simulink model "controller_Delta3D_feedback"  (R2018b)
settings: Solver=ode45  StartTime=0.0  StopTime=0.5  RelTol=1e-3  EnableMultiTasking=on
values from neighbouring files (symbols this model uses):
  g = 9.81    [project_week_5.m]
  h0 = thetaA_0(1)    [project_week_5.m]
  hm = thetaA_0(1)*0.5    [project_week_5.m]
  I_lower_xx = I_C(4)    [calculate_lagrange.m]    (also in calculate_lagrange_dependent.m; calculate_lagrange_fast.m; project_week_5.m = (1/12)*m_l*L(2)^2)
  I_lower_yy = I_C(5)    [calculate_lagrange.m]    (also in calculate_lagrange_dependent.m; calculate_lagrange_fast.m; project_week_5.m = (1/12)*m_l*L(2)^2)
  I_lower_zz = I_C(6)    [calculate_lagrange.m]    (also in calculate_lagrange_dependent.m; calculate_lagrange_fast.m; project_week_5.m = I_lower_xx/10)
  I_upper_xx = I_C(1)    [calculate_lagrange.m]    (also in calculate_lagrange_dependent.m; calculate_lagrange_fast.m; project_week_5.m = (1/12)*m_u*L(1)^2)
  I_upper_yy = I_C(2)    [calculate_lagrange.m]    (also in calculate_lagrange_dependent.m; calculate_lagrange_fast.m; project_week_5.m = (1/12)*m_u*L(1)^2)
  I_upper_zz = I_C(3)    [calculate_lagrange.m]    (also in calculate_lagrange_dependent.m; calculate_lagrange_fast.m; project_week_5.m = I_upper_xx/10)
  kc = M*wc^2*sqrt(alpha)    [project_week_5.m]
  L = [0.5,1,0.3,0.8]    [plot_inverse.m]    (also in project_week_5.m; project_week_5_boundaries.m = [0.8,1,0.4,0.5]; project_week_5_symbolic.m = [L_u L_l L_e L_b])
  m_l = 0.35    [project_week_5.m]
  m_p = 1    [project_week_5.m]
  m_u = 0.35    [project_week_5.m]
  q0d = q0(ind_d)    [project_week_5.m]
  q0i = q0(ind_i)    [project_week_5.m]
  R_L1_0 = R_L1_t(:,:,1)    [calculate_acceleration.m]    (also in calculate_position.m = R_L0(:,:,1); calculate_position_dep.m = R_L0(:,:,1); calculate_position_fast.m = R_L0(:,:,1); plot_inverse.m = R_A1*rot3D_Rodrigues([0;1;0],thetaL1_y_0))
  R_L2_0 = R_L2_t(:,:,1)    [calculate_acceleration.m]    (also in calculate_position.m = R_L0(:,:,2); calculate_position_dep.m = R_L0(:,:,2); calculate_position_fast.m = R_L0(:,:,2); plot_inverse.m = R_A2*rot3D_Rodrigues([0;1;0],thetaL2_y_0))
  R_L3_0 = R_L3_t(:,:,1)    [calculate_acceleration.m]    (also in calculate_position.m = R_L0(:,:,3); calculate_position_dep.m = R_L0(:,:,3); calculate_position_fast.m = R_L0(:,:,3); plot_inverse.m = R_A3*rot3D_Rodrigues([0;1;0],thetaL3_y_0))
  thetaA_0 = [thetaU1_y_0 ; thetaU2_y_0 ;thetaU3_y_0]    [plot_inverse.m]    (also in project_week_5.m; project_week_5_boundaries.m)
  ti = beta*tz    [project_week_5.m]
  tm = cycleTime    (= 0.35)    [project_week_5.m]
  tp = alpha*tz    [project_week_5.m]
  tz = 1/(wc*sqrt(alpha))    [project_week_5.m]
settings Model: Creator=wouterh  LastModifiedBy=sinai
settings DataIOCC: LimitDataPoints=on  SaveFormat=Array  SignalLoggingSaveFormat=ModelDataLogs
settings OptimizationCC: ExpressionDepthLimit=2147483647  InitFltsAndDblsToZero=on  LifeSpan=inf
settings DebuggingCC: UnderspecifiedInitializationDetection=Classic  MergeDetectMultiDrivingBlocksExec=none  SolverPrmCheckMsg=warning  FcnCallInpInsideContextMsg=warning  StateNameClashWarn=warning  LibraryContextMissingDiagnostic=none  SFUnexpectedBacktrackingDiag=warning  SFNoUnconditionalDefaultTransitionDiag=warning  SFExecutionAtInitializationDiag=none
settings HardwareCC: ProdBitPerPointer=32  ProdBitPerSizeT=32  ProdBitPerPtrDiffT=32  ProdLargestAtomicFloat=None  ProdIntDivRoundTo=Undefined  ProdEndianess=Unspecified  ProdWordSize=32  ProdHWDeviceType=32-bit Generic
settings ModelReferenceCC: PropagateSignalLabelsOutOfModel=off
settings SFSimCC: SimUseLocalCustomCode=off
settings RTWCC: RTWUseLocalCustomCode=off
settings CodeAppCC: StateflowObjectComments=on
settings GRTTargetCC: TargetLangStandard=C89/C90 (ANSI)  CombineOutputUpdateFcns=off  GRTInterface=on
settings ConfigComp: CovMetricSettings=dw  CovHtmlReporting=on  CovSaveCumulativeToWorkspaceVar=on  CovSaveSingleToWorkspaceVar=on  CovExternalEMLEnable=off

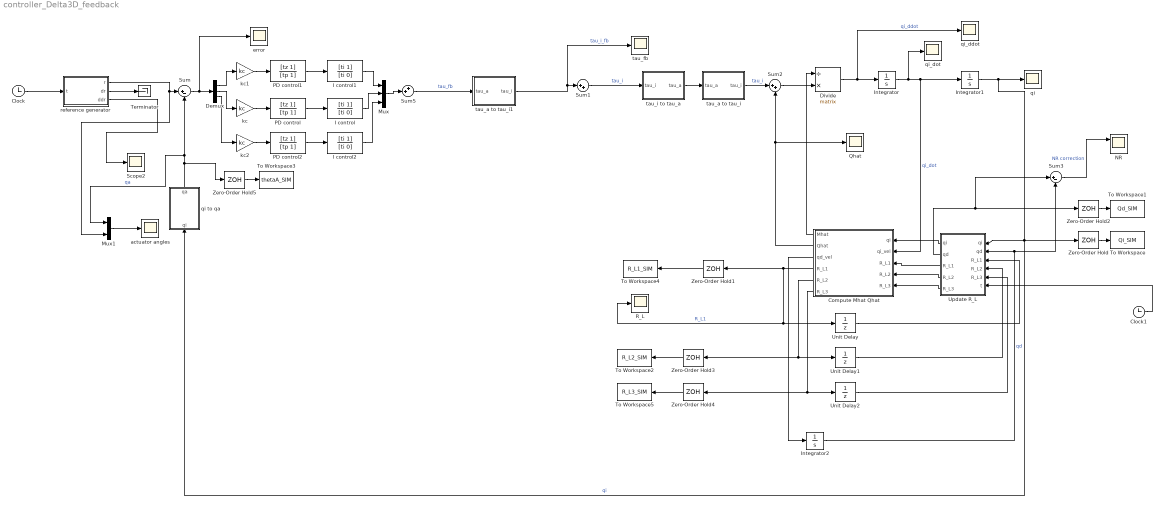
== system controller_Delta3D_feedback ==
  Clock : Clock
  Clock1 : Clock
  Compute Mhat Qhat : MATLAB Function  TreatAsAtomicUnit=on
  Demux : Demux  Outputs=3
  Divide : Product  Inputs=/*  Multiplication=Matrix(*)
  I control : TransferFcn  Numerator=[ti 1]  Denominator=[ti 0]
  I control1 : TransferFcn  Numerator=[ti 1]  Denominator=[ti 0]
  I control2 : TransferFcn  Numerator=[ti 1]  Denominator=[ti 0]
  Integrator : Integrator
  Integrator1 : Integrator  InitialCondition=q0i
  Integrator2 : Integrator  InitialCondition=q0d
  Mux : Mux  Inputs=3
  Mux1 : Mux  Inputs=2
  NR : Scope  NumInputPorts=2
  PD control : TransferFcn  Numerator=[tz 1]  Denominator=[tp 1]
  PD control1 : TransferFcn  Numerator=[tz 1]  Denominator=[tp 1]
  PD control2 : TransferFcn  Numerator=[tz 1]  Denominator=[tp 1]
  Qhat : Scope
  R_L : Scope
  Scope2 : Scope
  Sum : Sum  Inputs=|+-
  Sum1 : Sum  Inputs=|++
  Sum2 : Sum  Inputs=|++
  Sum3 : Sum  Inputs=|+-
  Sum5 : Sum  Inputs=++|
  Terminator : Terminator
  To Workspace : ToWorkspace  VariableName=Qi_SIM  SaveFormat=Timeseries  SampleTime=-1
  To Workspace1 : ToWorkspace  VariableName=Qd_SIM  SaveFormat=Timeseries  SampleTime=-1
  To Workspace2 : ToWorkspace  VariableName=R_L2_SIM  SaveFormat=Timeseries  SampleTime=-1
  To Workspace3 : ToWorkspace  VariableName=thetaA_SIM  SaveFormat=Timeseries  SampleTime=-1
  To Workspace4 : ToWorkspace  VariableName=R_L1_SIM  SaveFormat=Timeseries  SampleTime=-1
  To Workspace5 : ToWorkspace  VariableName=R_L3_SIM  SaveFormat=Timeseries  SampleTime=-1
  Unit Delay : UnitDelay  InitialCondition=R_L1_0  SampleTime=-1
  Unit Delay1 : UnitDelay  InitialCondition=R_L2_0  SampleTime=-1
  Unit Delay2 : UnitDelay  InitialCondition=R_L3_0  SampleTime=-1
  Update R_L : MATLAB Function  TreatAsAtomicUnit=on  SystemSampleTime=0.001
  Zero-Order Hold{,1..5} (6 alike) : ZeroOrderHold  SampleTime=0.02
  actuator angles : Scope
  error : Scope
  kc : Gain  Gain=kc
  kc1 : Gain  Gain=kc
  kc2 : Gain  Gain=kc
  qi : Scope
  qi to qa : MATLAB Function  TreatAsAtomicUnit=on
  qi_ddot : Scope
  qi_dot : Scope
  reference generator : MATLAB Function  TreatAsAtomicUnit=on
  tau_a to tau_i : MATLAB Function  TreatAsAtomicUnit=on
  tau_a to tau_i1 : MATLAB Function  TreatAsAtomicUnit=on
  tau_fb : Scope
  tau_i to tau_a : MATLAB Function  TreatAsAtomicUnit=on
  wires:
  Clock/1 -> reference generator/1(t)
  reference generator/2(dr) -> Terminator/1
  reference generator/3(ddr) -> Scope2/1
  Sum/1 -> Demux/1, error/1
  PD control/1 -> I control/1
  Divide/1 -> qi_ddot/1, Integrator/1  "qi_ddot"
  Integrator/1 -> qi_dot/1, Integrator1/1, Compute Mhat Qhat/2(qi_vel)  "qi_dot"
  Integrator1/1 -> qi to qa/1(qi), Update R_L/1("qi "), Zero-Order Hold/1, qi/1  "qi"
  Compute Mhat Qhat/1(Mhat) -> Divide/1
  PD control1/1 -> I control1/1
  I control/1 -> Mux/2
  I control1/1 -> Mux/1
  Mux/1 -> Sum5/2
  Sum5/1 -> tau_a to tau_i1/1(tau_a)  "tau_fb"
  Mux1/1 -> actuator angles/1
  Compute Mhat Qhat/3(qd_vel) -> Integrator2/1
  kc1/1 -> PD control1/1
  Demux/1 -> kc1/1
  Demux/2 -> kc/1
  kc/1 -> PD control/1
  reference generator/1(r) -> Mux1/2, Sum/1
  Zero-Order Hold/1 -> To Workspace/1
  Zero-Order Hold2/1 -> To Workspace1/1
  Unit Delay/1 -> Update R_L/3("R_L1 ")
  Compute Mhat Qhat/4(R_L1) -> Zero-Order Hold1/1, R_L/1, Unit Delay/1  "R_L1"
  I control2/1 -> Mux/3
  kc2/1 -> PD control2/1
  PD control2/1 -> I control2/1
  Demux/3 -> kc2/1
  Sum2/1 -> Divide/2
  tau_a to tau_i/1(tau_i) -> Sum2/1  "tau_i"
  qi to qa/1(qa) -> Mux1/1, Sum/2, Zero-Order Hold5/1  "qa"
  Compute Mhat Qhat/5(R_L2) -> Zero-Order Hold3/1, Unit Delay1/1
  Compute Mhat Qhat/6(R_L3) -> Unit Delay2/1, Zero-Order Hold4/1
  Unit Delay2/1 -> Update R_L/5("R_L3 ")
  tau_i to tau_a/1(tau_a) -> tau_a to tau_i/1(tau_a)
  Sum1/1 -> tau_i to tau_a/1(tau_i)  "tau_i"
  tau_a to tau_i1/1(tau_i) -> tau_fb/1, Sum1/1  "tau_i_fb"
  Unit Delay1/1 -> Update R_L/4("R_L2 ")
  Zero-Order Hold1/1 -> To Workspace4/1
  Zero-Order Hold3/1 -> To Workspace2/1
  Update R_L/1(qi) -> Compute Mhat Qhat/1(qi)
  Integrator2/1 -> Sum3/2, Update R_L/2("qd ")  "qd"
  Update R_L/2(qd) -> Sum3/1, Zero-Order Hold2/1
  Update R_L/3(R_L1) -> Compute Mhat Qhat/3("R_L1 ")
  Update R_L/4(R_L2) -> Compute Mhat Qhat/4("R_L2 ")
  Update R_L/5(R_L3) -> Compute Mhat Qhat/5("R_L3 ")
  Zero-Order Hold4/1 -> To Workspace5/1
  Clock1/1 -> Update R_L/6(t)
  Zero-Order Hold5/1 -> To Workspace3/1
  Sum3/1 -> NR/1  "NR correction"
  Compute Mhat Qhat/2(Qhat) -> Qhat/1, Sum2/2

== matlab function controller_Delta3D_feedback/Compute Mhat Qhat ==
  data: qi input; qi_vel input; R_L1 input; R_L2 input; R_L3 input; Mhat output; Qhat output; m_u parameter; m_p parameter; m_l parameter; L parameter; g parameter; I_upper_xx parameter; I_upper_yy parameter; I_upper_zz parameter; I_lower_xx parameter; I_lower_yy parameter; I_lower_zz parameter; thetaA_0 parameter; qd_vel output; R_L1 output; R_L2 output; R_L3 output
function [Mhat, Qhat,qd_vel,R_L1,R_L2,R_L3] = ...
    computeMhatQhat(qi,qi_vel,R_L1,R_L2,R_L3,...
        m_u, m_p, m_l, L, g,...
        I_upper_xx, I_upper_yy, I_upper_zz,...
        I_lower_xx, I_lower_yy, I_lower_zz,...
        thetaA_0)
% Compute dynamics for the system 
% Assume the model is perfect, so this is a copy past of M_Q_AC_model

%Pre-initialise for Simulink
Mhat=zeros(9,9);
Qhat=zeros(9,1);
qd_vel=zeros(33,1);

% independent and dependent co-ordinate indices
ind_i=[7:9,19:21,31:33]';
% ind_d=(1:42)'; 
% ind_d(ind_i)=[]; % remove independent co-ordinates -> doesn't work in Simulink
ind_d = [1:6,10:18,22:30,34:42]';

%% Parameters
L_u=L(1);
L_l=L(2);
L_e=L(3);
L_b=L(4);

thetaA1 = qi(1)/(+3^(1/2)/2) + thetaA_0(1); 
thetaA2 = qi(4)/(-3^(1/2)/2) + thetaA_0(2); 
thetaA3 = qi(8); 
   
% upper rotation matrices
R_A1=rot3D_Rodrigues([0;0;1],-2*pi/3); % constant
R_U1=R_A1*rot3D_Rodrigues([0;1;0],thetaA1); 

R_A2=rot3D_Rodrigues([0;0;1],2*pi/3); % constant
R_U2=R_A2*rot3D_Rodrigues([0;1;0],thetaA2); 

R_A3=rot3D_Rodrigues([0;0;1],0); % constant
R_U3=R_A3*rot3D_Rodrigues([0;1;0],thetaA3); 

% R_L1
rL1_1_1 = R_L1(1,1); rL1_1_2 = R_L1(1,2); rL1_1_3 = R_L1(1,3);
rL1_2_1 = R_L1(2,1); rL1_2_2 = R_L1(2,2); rL1_2_3 = R_L1(2,3);
rL1_3_1 = R_L1(3,1); rL1_3_2 = R_L1(3,2); rL1_3_3 = R_L1(3,3);

% R_L2
rL2_1_1 = R_L2(1,1); rL2_1_2 = R_L2(1,2); rL2_1_3 = R_L2(1,3);
rL2_2_1 = R_L2(2,1); rL2_2_2 = R_L2(2,2); rL2_2_3 = R_L2(2,3);
rL2_3_1 = R_L2(3,1); rL2_3_2 = R_L2(3,2); rL2_3_3 = R_L2(3,3);

% R_L3
rL3_1_1 = R_L3(1,1); rL3_1_2 = R_L3(1,2); rL3_1_3 = R_L3(1,3);
rL3_2_1 = R_L3(2,1); rL3_2_2 = R_L3(2,2); rL3_2_3 = R_L3(2,3);
rL3_3_1 = R_L3(3,1); rL3_3_2 = R_L3(3,2); rL3_3_3 = R_L3(3,3);

%% Calculate moment inertias in the inertia frame
I_U1=R_U1*diag([I_upper_xx,I_upper_yy I_upper_zz])*R_U1.';
I_U2=R_U2*diag([I_upper_xx,I_upper_yy I_upper_zz])*R_U2.';
I_U3=R_U3*diag([I_upper_xx,I_upper_yy I_upper_zz])*R_U3.';

I_L1=R_L1*diag([I_lower_xx,I_lower_yy I_lower_zz])*R_L1.';
I_L2=R_L2*diag([I_lower_xx,I_lower_yy I_lower_zz])*R_L2.';
I_L3=R_L3*diag([I_lower_xx,I_lower_yy I_lower_zz])*R_L3.';

%% Partition into M*Qddot=[Mdd Mdi; Mid Mii]*[Qi_ddot Qd_ddot]
Mii = [I_U1 zeros(3,6);
      zeros(3,3) I_U2  zeros(3,3);
      zeros(3,6) I_U3];
Mdd = diag([0 0 0 ...
           m_u*[1 1 1]              ...
           m_l*[1 1 1] I_lower_xx I_lower_yy I_lower_zz ...
           m_u*[1 1 1]              ...
           m_l*[1 1 1] I_lower_xx I_lower_yy I_lower_zz ...
           m_u*[1 1 1]              ...
           m_l*[1 1 1] I_lower_xx I_lower_yy I_lower_zz ...
           m_p*[1 1 1] ]); 
% Correct Mdd
Mdd(10:12,10:12)=I_L1;
Mdd(19:21,19:21)=I_L2;
Mdd(28:30,28:30)=I_L3;
  
Mdi = zeros(33,9);
Mid = zeros(9,33);

Jacobian_d = Jacobian_dNumeric(L_l,...
                               rL1_1_1,rL1_1_2,...%R_L1
                               rL1_2_1,rL1_2_2,...
                               rL1_3_1,rL1_3_2,...
                               rL2_1_1,rL2_1_2,...%R_L2
                               rL2_2_1,rL2_2_2,...
                               rL2_3_1,rL2_3_2,...
                               rL3_1_1,rL3_1_2,...%R_L3
                               rL3_2_1,rL3_2_2,...
                               rL3_3_1,rL3_3_2);
Jacobian_i = Jacobian_iNumeric(L_u,thetaA1,thetaA2,thetaA3);

%% Compute dependent velocities
J = Jacobian_d\Jacobian_i;
qd_vel = -J*qi_vel;

%match symbolic variables to numeric variables
qvel=zeros(42,1);
qvel(ind_i)=qi_vel;
qvel(ind_d)=qd_vel;

qvel1=qvel(1);qvel2=qvel(2);qvel3=qvel(3);
qvel4=qvel(4);qvel5=qvel(5);qvel6=qvel(6);
qvel7=qvel(7);qvel8=qvel(8);qvel9=qvel(9);
qvel10=qvel(10);qvel11=qvel(11);qvel12=qvel(12);
qvel13=qvel(13);qvel14=qvel(14);qvel15=qvel(15);
qvel16=qvel(16);qvel17=qvel(17);qvel18=qvel(18);
qvel19=qvel(19);qvel20=qvel(20);qvel21=qvel(21);
qvel22=qvel(22);qvel23=qvel(23);qvel24=qvel(24);
qvel25=qvel(25);qvel26=qvel(26);qvel27=qvel(27);
qvel28=qvel(28);qvel29=qvel(29);qvel30=qvel(30);
qvel31=qvel(31);qvel32=qvel(32);qvel33=qvel(33);
qvel34=qvel(34);qvel35=qvel(35);qvel36=qvel(36);
qvel37=qvel(37);qvel38=qvel(38);qvel39=qvel(39);
qvel40=qvel(40);qvel41=qvel(41);qvel42=qvel(42);

Gamma_without_driving = Gamma_without_drivingNumeric(...
    L_l,L_u,...
    qvel7,qvel8,qvel9,...
    qvel13,qvel14,qvel15,...
    qvel19,qvel20,qvel21,...
    qvel25,qvel26,qvel27,...
    qvel31,qvel32,qvel33,...
    qvel37,qvel38,qvel39,...
    rL1_1_1,rL1_1_2,...%R_L1
    rL1_2_1,rL1_2_2,...
    rL1_3_1,rL1_3_2,...
    rL2_1_1,rL2_1_2,...%R_L2
    rL2_2_1,rL2_2_2,...
    rL2_3_1,rL2_3_2,...
    rL3_1_1,rL3_1_2,...%R_L3
    rL3_2_1,rL3_2_2,...
    rL3_3_1,rL3_3_2,...
    thetaA1,thetaA2,thetaA3);

%% Compute Q_Ai and Q_Ad
Q_Ad=zeros(33,1);
% Gravity
Q_Ad(6)=-m_u*g;
Q_Ad(9)=-m_l*g;
Q_Ad(15)=-m_u*g;
Q_Ad(18)=-m_l*g;
Q_Ad(24)=-m_u*g;
Q_Ad(27)=-m_l*g;
Q_Ad(33)=-m_p*g;

% Calculate gyroscopic forces in the inertia frame
C_U1=tilde(qvel(7:9))*  I_U1*qvel(7:9);
C_U2=tilde(qvel(19:21))*I_U2*qvel(19:21);
C_U3=tilde(qvel(31:33))*I_U3*qvel(31:33);

C_L1=tilde(qvel(13:15))*I_L1*qvel(13:15);
C_L2=tilde(qvel(25:27))*I_L2*qvel(25:27);
C_L3=tilde(qvel(37:39))*I_L3*qvel(37:39);
% dependent C, lower angles
Q_Ad(10:12)=Q_Ad(10:12)-C_L1;  
Q_Ad(19:21)=Q_Ad(19:21)-C_L2;
Q_Ad(28:30)=Q_Ad(28:30)-C_L3;

% independent C
Q_Ai=zeros(9,1);
Q_Ai(1:3)=Q_Ai(1:3)-C_U1;
Q_Ai(4:6)=Q_Ai(4:6)-C_U2;
Q_Ai(7:9)=Q_Ai(7:9)-C_U3;
%% Compute Ouputs
J2 = Jacobian_d\Gamma_without_driving;

Mhat = Mii - Mid*J - J.'*(Mdi - Mdd*J); 
Qhat = Q_Ai-Mid*J2 -(J.')*(Q_Ad -Mdd*J2);

end

== matlab function controller_Delta3D_feedback/Update R_L ==
  data: qi input; qi output; qd input; qd output; L parameter; R_L1 input; R_L2 input; R_L3 input; R_L1 output; R_L1_0 parameter; R_L2_0 parameter; R_L3_0 parameter; thetaA_0 parameter; R_L2 output; R_L3 output; t input
function [qi,qd,R_L1,R_L2,R_L3] = fcn(qi,qd,L, R_L1,R_L2,R_L3,R_L1_0, R_L2_0, R_L3_0, thetaA_0,t)
% Compute dynamics for the system 
% Assume the model is perfect, so this is a copy past of M_Q_AC_model
% Requires running Project_week_4 first to get Mhat and Qhat
% IMPORTANT: the sample time of this block MUST be set to a finite value.
%            That is, not -1 for inherited
%            This sample time determines the period the lower angles have an
%            approximately constant omega

%Pre-initialise for Simulink
L_u=L(1);
L_l=L(2);
L_e=L(3);
L_b=L(4);
tolerance=0.0001;


thetaA1 = qi(1)/(+3^(1/2)/2) + thetaA_0(1); %qi()=thetaU1_x
thetaA2 = qi(4)/(-3^(1/2)/2) + thetaA_0(2); %qi()=thetaU2_x
thetaA3 = qi(8);                            %qi()=thetaU3_y

% upper rotation matrices
R_A1=rot3D_Rodrigues([0;0;1],-2*pi/3); % constant
R_U1=R_A1*rot3D_Rodrigues([0;1;0],thetaA1); 

R_A2=rot3D_Rodrigues([0;0;1],2*pi/3); % constant
R_U2=R_A2*rot3D_Rodrigues([0;1;0],thetaA2); 

R_A3=rot3D_Rodrigues([0;0;1],0); % constant
R_U3=R_A3*rot3D_Rodrigues([0;1;0],thetaA3); 

newton_iterations = 0;
S=ones(33,1)*tolerance;
while norm(S) > tolerance
    newton_iterations = newton_iterations +1;
    
    % Match symbols to numeric values
    M_x = qd(1);  M_y = qd(2);  M_z = qd(3);
    U1_x = qd(4); U1_y = qd(5); U1_z = qd(6);
    L1_x = qd(7); L1_y = qd(8); L1_z = qd(9);
 thetaL1_x = qd(10); thetaL1_y = qd(11); thetaL1_z = qd(12);
    U2_x = qd(13); U2_y = qd(14); U2_z = qd(15);
    L2_x = qd(16); L2_y = qd(17); L2_z = qd(18);
 thetaL2_x = qd(19); thetaL2_y = qd(20); thetaL2_z = qd(21);
    U3_x = qd(22); U3_y = qd(23); U3_z = qd(24);
    L3_x = qd(25); L3_y = qd(26); L3_z = qd(27);
 thetaL3_x = qd(28); thetaL3_y = qd(29); thetaL3_z = qd(30);
    P_x = qd(31);   P_y = qd(32);  P_z = qd(33);
    
    % R_L1
    rL1_1_1 = R_L1(1,1); rL1_1_2 = R_L1(1,2); rL1_1_3 = R_L1(1,3);
    rL1_2_1 = R_L1(2,1); rL1_2_2 = R_L1(2,2); rL1_2_3 = R_L1(2,3);
    rL1_3_1 = R_L1(3,1); rL1_3_2 = R_L1(3,2); rL1_3_3 = R_L1(3,3);

    % R_L2
    rL2_1_1 = R_L2(1,1); rL2_1_2 = R_L2(1,2); rL2_1_3 = R_L2(1,3);
    rL2_2_1 = R_L2(2,1); rL2_2_2 = R_L2(2,2); rL2_2_3 = R_L2(2,3);
    rL2_3_1 = R_L2(3,1); rL2_3_2 = R_L2(3,2); rL2_3_3 = R_L2(3,3);

    % R_L3
    rL3_1_1 = R_L3(1,1); rL3_1_2 = R_L3(1,2); rL3_1_3 = R_L3(1,3);
    rL3_2_1 = R_L3(2,1); rL3_2_2 = R_L3(2,2); rL3_2_3 = R_L3(2,3);
    rL3_3_1 = R_L3(3,1); rL3_3_2 = R_L3(3,2); rL3_3_3 = R_L3(3,3);
    
    %S = subs(System,[Q_sym],[q]);
    S = [...
    ... # Arm 1:  3x3 = 9 constraints
    [M_x;M_y;M_z] + R_A1*[L(4)/2; 0 ;0] - [U1_x; U1_y; U1_z] - R_U1*[0;0;L(1)/2];
    [U1_x; U1_y; U1_z] + R_U1*[0;0;-L(1)/2] - [L1_x; L1_y; L1_z] - R_L1*[0;0;L(2)/2];
    [L1_x; L1_y; L1_z] + R_L1*[0;0;-L(2)/2] - [P_x; P_y; P_z] - R_A1*[L(3)/2;0 ;0];
    ... # Arm 2:  3x3 = 9 constraints
    [M_x;M_y;M_z] + R_A2*[L(4)/2; 0 ;0] - [U2_x; U2_y; U2_z] - R_U2*[0;0;L(1)/2];
    [U2_x; U2_y; U2_z] + R_U2*[0;0;-L(1)/2] - [L2_x; L2_y; L2_z] - R_L2*[0;0;L(2)/2];
    [L2_x; L2_y; L2_z] + R_L2*[0;0;-L(2)/2] - [P_x; P_y; P_z] - R_A2*[L(3)/2;0 ;0];
    ... # Arm 3:  3x3 = 9 constraints
    [M_x;M_y;M_z] + R_A3*[L(4)/2; 0 ;0] - [U3_x; U3_y; U3_z] - R_U3*[0;0;L(1)/2];
    [U3_x; U3_y; U3_z] + R_U3*[0;0;-L(1)/2] - [L3_x; L3_y; L3_z] - R_L3*[0;0;L(2)/2];
    [L3_x; L3_y; L3_z] + R_L3*[0;0;-L(2)/2] - [P_x; P_y; P_z] - R_A3*[L(3)/2;0 ;0];
        ... # Fixed variables:  3 constraints
    [M_x;M_y;M_z];
     ... # Fixed lower link spin in own axis
    [0 1 0]*R_L1.'*R_L1_0*[1;0;0];  % L1_y has no component in L1_x_0
    [0 1 0]*R_L2.'*R_L2_0*[1;0;0]; % L2_y has no component in L2_x_0
    [0 1 0]*R_L3.'*R_L3_0*[1;0;0]; % L3_y has no component in L3_x_0
    ];

   Jacobian_d = Jacobian_dNumeric(L_l,...
                               rL1_1_1,rL1_1_2,...%R_L1
                               rL1_2_1,rL1_2_2,...
                               rL1_3_1,rL1_3_2,...
                               rL2_1_1,rL2_1_2,...%R_L2
                               rL2_2_1,rL2_2_2,...
                               rL2_3_1,rL2_3_2,...
                               rL3_1_1,rL3_1_2,...%R_L3
                               rL3_2_1,rL3_2_2,...
                               rL3_3_1,rL3_3_2);
    Delta = -Jacobian_d\S;
    qd = qd+Delta;  % if use q=q-Delta, the calculate_position.m code no longer works 
    % Update the Rotation matrices using a first approximation of the
    % Rodriguez formula
                      % Delta theta_L
%     deltaR1=eye(3)+tilde(Delta(10:12));
%     deltaR2=eye(3)+tilde(Delta(19:21));
%     deltaR3=eye(3)+tilde(Delta(28:30));
    deltaR1=expm(tilde(Delta(10:12)));
    deltaR2=expm(tilde(Delta(19:21)));
    deltaR3=expm(tilde(Delta(28:30)));
    R_L1=deltaR1*R_L1;
    R_L2=deltaR2*R_L2;
    R_L3=deltaR3*R_L3;
    
end


end

== matlab function controller_Delta3D_feedback/tau_a to tau_i ==
  data: tau_a input; tau_i output
function tau_i = fcn(tau_a)
% convert independent torques to actuator torques
% implicient input R_U, where thetaU1_z_0=-2*pi/3 and thetaU2_z_0=+2*pi/3

% JacobianA_a =[ 3^(1/2)/2, -0.5, 0,   0, 0, 0, 0, 0, 0;
%                0, 0, 0,  -3^(1/2)/2, -0.5, 0, 0, 0, 0;
%                0, 0, 0,              0, 0, 0, 0, 1, 0];

%tau_i= JacobianA_a'*tau_a;

tau_i=tau_a;

end

== matlab function controller_Delta3D_feedback/tau_i to tau_a ==
  data: tau_i input; tau_a output
function tau_a = fcn(tau_i)
% convert actuator torques to independent torques
% implicient input R_U, where thetaU1_z_0=-2*pi/3 and thetaU2_z_0=+2*pi/3

% JacobianA_a =[ 3^(1/2)/2, -0.5, 0,   0, 0, 0, 0, 0, 0;
%                0, 0, 0,  -3^(1/2)/2, -0.5, 0, 0, 0, 0;
%                0, 0, 0,              0, 0, 0, 0, 1, 0];

%tau_a= JacobianA_a*tau_i;

tau_a=tau_i;
end

== matlab function controller_Delta3D_feedback/qi to qa ==
  data: qi input; qa output; thetaA_0 parameter
function qa = fcn(qi,thetaA_0)
% convert independent co-ordinates to actuator co-ordinates
% implicient input R_U, where thetaU1_z_0=-2*pi/3 and thetaU2_z_0=+2*pi/3

qa=zeros(3,1);

thetaA1 = qi(1)/(+3^(1/2)/2) + thetaA_0(1); %qi()=thetaU1_x
thetaA2 = qi(4)/(-3^(1/2)/2) + thetaA_0(2); %qi()=thetaU2_x
thetaA3 = qi(8);                            %qi()=thetaU3_y

qa(1)=thetaA1;
qa(2)=thetaA2;
qa(3)=thetaA3;

end

== matlab function controller_Delta3D_feedback/reference generator ==
  data: t input; r output; dr output; ddr output; hm parameter; tm parameter; h0 parameter
function [r,dr,ddr] = ref(t, hm, tm, h0)
% create a skew-sine motion profile


if t < tm
    r   = h0+hm/tm*t-hm/(2*pi)   *sin(2*pi/tm*t);
    dr  =    hm/tm  -hm/tm       *cos(2*pi/tm*t);
    ddr =           +hm/tm^2*2*pi*sin(2*pi/tm*t);
else
    r   = h0+hm;
    dr  = 0*hm/tm;
    ddr = 0*hm/tm^2;
end

r=h0;

== matlab function controller_Delta3D_feedback/tau_a to tau_i1 ==
  data: tau_a input; tau_i output
function tau_i = fcn(tau_a)
% convert independent torque to actuator torque
% implicient input R_U, where thetaU1_z_0=-2*pi/3 and thetaU2_z_0=+2*pi/3

JacobianA_a =[ (3^(1/2)/2), (-0.5), 0 0, 0, 0,  0, 0, 0;
               0, 0, 0, (-3^(1/2)/2),(-0.5), 0,  0, 0, 0;
               0, 0, 0,       0, 0, 0,               0, 1, 0];


tau_i=JacobianA_a.'*tau_a;

end
